simulink model "simulate"  (R2020a)
settings: Solver=VariableStepAuto  StartTime=0.0  StopTime=10  RelTol=1e-3
values from neighbouring files (symbols this model uses):
  A = [0, 1; g/L, 0]    [main.m]    (also in plant.m = [0, 1; -g/L, 0])
  B = [0; 1/(m * L^2)]    [main.m]    (also in plant.m = [0; 1/m])
  C = [1, 0]    [main.m]    (also in plant.m)
settings Model: Creator=Takumi  LastModifiedBy=Takumi

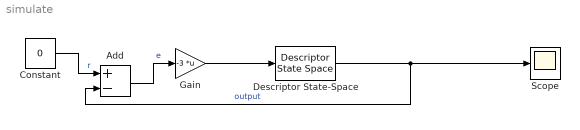
== system simulate ==
  Add : Sum  Inputs=+-
  Constant : Constant  Value=0
  Descriptor State-Space : DescriptorStateSpace  E=eye(2)  A=A  B=B  C=C  D=0  InitialCondition=0.1
  Gain : Gain  Gain=-3  Multiplication=Matrix(K*u) (u vector)
  Scope : Scope
  wires:
  Descriptor State-Space/1 -> Add/2, Scope/1  "output"
  Gain/1 -> Descriptor State-Space/1
  Constant/1 -> Add/1  "r"
  Add/1 -> Gain/1  "e"
